simulink model "controllerB_2013B"  (R2013b)
settings: Solver=ode45  StartTime=0.0  StopTime=sim_run  FixedStep=0.001  RelTol=1e-3
InitFcn:
  | zh = 0.01;
undefined symbols (not defined in the file): Standard_Devices, UDP_Protocol, zh_step
libraries: simulink x2, rtwinlib x2, dspnetwork x2
settings Model: Creator=Lenka  LastModifiedBy=Anony
settings DebuggingCC: UnderspecifiedInitializationDetection=Simplified  MergeDetectMultiDrivingBlocksExec=error  FrameProcessingCompatibilityMsg=error
settings GRTTargetCC: CodeReplacementLibrary=C89/C90 (ANSI)

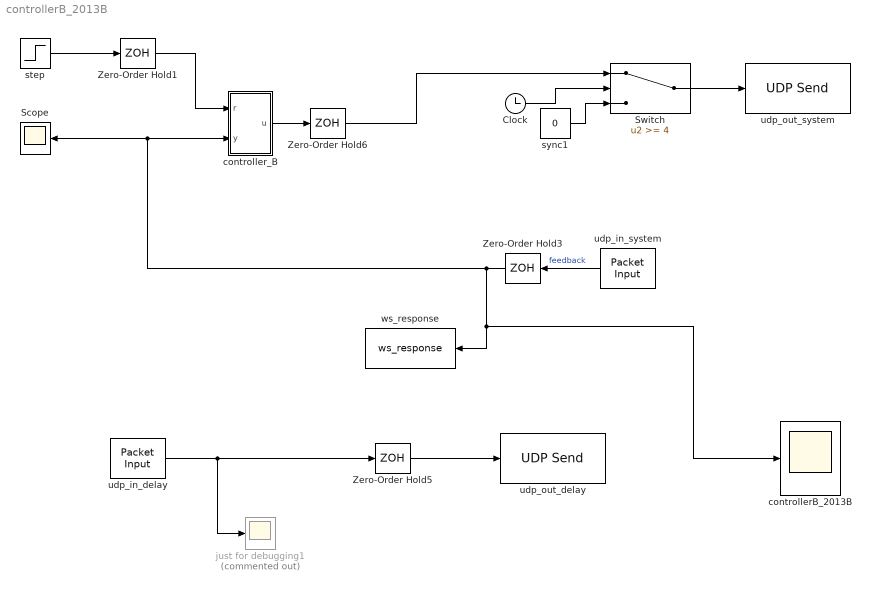
== system controllerB_2013B ==
  Clock : Clock
  Scope : Scope
      settings: YMin=-10  YMax=10
  Switch : Switch  Threshold=4
  Zero-Order Hold{1,3,5..6} (4 alike) : ZeroOrderHold  SampleTime=zh_step
  controllerB_2013B : Scope
      settings: YMin=-1.00000  YMax=1.00000
  controller_B : Subsystem
  just for debugging1 : Scope  Commented=on
      settings: YMin=-10  YMax=10
  step : Step  After=0.15  SampleTime=0
  sync1 : Constant  Value=0
  udp_in_delay : rtwinlib/Packet Input  SampleTime=0.001  MaxMissedTicks=inf  ShowMissedTicks=off  YieldWhenWaiting=off  DrvName=Standard_Devices/UDP_Protocol  DrvAddress=21000  DrvOptions=[2468394757 21000]  PacketSize=8  DataTypes='double'  ShowReady=off  ShowError=off  PacketID=1  ByteOrder=1  ShowTimestamp=off
      settings: AttributesFormatString=Standard Devices\nUDP Protocol [6982h]
  udp_in_system : rtwinlib/Packet Input  SampleTime=0.001  MaxMissedTicks=inf  ShowMissedTicks=off  YieldWhenWaiting=off  DrvName=Standard_Devices/UDP_Protocol  DrvAddress=21500  DrvOptions=[2468394757 21500]  PacketSize=8  DataTypes='double'  ShowReady=off  ShowError=off  PacketID=1  ByteOrder=1  ShowTimestamp=off
      settings: AttributesFormatString=Standard Devices\nUDP Protocol [6F54h]
  udp_out_delay : dspnetwork/UDP Send  remoteURL='147.32.183.5'  remotePort=20000  localURL='0.0.0.0'  localPortSource=Automatically determine  localPort=27000  sampletime=-1  separateLengthPort=0
  udp_out_system : dspnetwork/UDP Send  remoteURL='147.32.183.5'  remotePort=20500  localURL='0.0.0.0'  localPortSource=Automatically determine  localPort=27000  sampletime=-1  separateLengthPort=0
  ws_response : ToWorkspace  VariableName=ws_response  SampleTime=zh_step  SaveFormat=Timeseries
  wires:
  step/1 -> Zero-Order Hold1/1
  udp_in_system/1 -> Zero-Order Hold3/1  "feedback"
  Zero-Order Hold3/1 -> controllerB_2013B/1, ws_response/1, controller_B/2(y), Scope/1
  Zero-Order Hold1/1 -> controller_B/1(r)
  controller_B/1(u) -> Zero-Order Hold6/1
  Switch/1 -> udp_out_system/1
  Zero-Order Hold6/1 -> Switch/1
  Clock/1 -> Switch/2
  sync1/1 -> Switch/3
  udp_in_delay/1 -> just for debugging1/1, Zero-Order Hold5/1
  Zero-Order Hold5/1 -> udp_out_delay/1

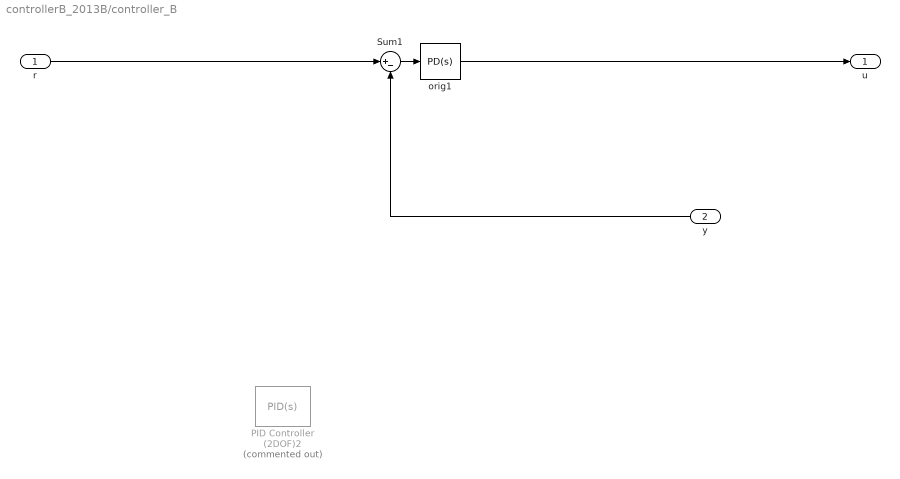
== system controllerB_2013B/controller_B ==
  r : Inport
  y : Inport  Port=2
  PID Controller (2DOF)2 : simulink/Continuous/PID Controller (2DOF)  Commented=on  Controller=PID  TimeDomain=Continuous-time  SampleTime=-1  IntegratorMethod=Forward Euler  FilterMethod=Forward Euler  Form=Parallel  P=6.3799380872686  I=2.12979603411331  D=3.6093223618413  N=48.5068620404972  b=2.39624043732871  c=0.716079145801974  InitialConditionSource=internal  InitialConditionForIntegrator=0  InitialConditionForFilter=0  ExternalReset=none  LimitOutput=off  UpperSaturationLimit=inf  LowerSaturationLimit=-inf  LinearizeAsGain=on  AntiWindupMode=none  Kb=1  TrackingMode=off  Kt=1  PParamMin=[]  PParamMax=[]  IParamMin=[]  IParamMax=[]  DParamMin=[]  DParamMax=[]  NParamMin=[]  NParamMax=[]  bParamMin=[]  bParamMax=[]  cParamMin=[]  cParamMax=[]  KbParamMin=[]  KbParamMax=[]  KtParamMin=[]  KtParamMax=[]  POutMin=[]  POutMax=[]  IOutMin=[]  IOutMax=[]  DOutMin=[]  DOutMax=[]  NOutMin=[]  NOutMax=[]  bOutMin=[]  bOutMax=[]  cOutMin=[]  cOutMax=[]  KbOutMin=[]  KbOutMax=[]  KtOutMin=[]  KtOutMax=[]  IntegratorOutMin=[]  IntegratorOutMax=[]  FilterOutMin=[]  FilterOutMax=[]  SumOutMin=[]  SumOutMax=[]  Sum1OutMin=[]  Sum1OutMax=[]  Sum2OutMin=[]  Sum2OutMax=[]  Sum3OutMin=[]  Sum3OutMax=[]  SumI1OutMin=[]  SumI1OutMax=[]  SumI2OutMin=[]  SumI2OutMax=[]  SumI3OutMin=[]  SumI3OutMax=[]  SumDOutMin=[]  SumDOutMax=[]  SaturationOutMin=[]  SaturationOutMax=[]  IntegratorContinuousStateAttributes=''  IntegratorStateMustResolveToSignalObject=off  IntegratorRTWStateStorageClass=Auto  FilterContinuousStateAttributes=''  FilterStateMustResolveToSignalObject=off  FilterRTWStateStorageClass=Auto
  Sum1 : Sum  Inputs=|+-
  orig1 : simulink/Continuous/PID Controller  Controller=PD  TimeDomain=Continuous-time  SampleTime=-1  IntegratorMethod=Forward Euler  FilterMethod=Forward Euler  Form=Parallel  P=0.0142  I=0.0175856984919557  D=0.0001  N=100  InitialConditionSource=internal  InitialConditionForIntegrator=0  InitialConditionForFilter=0  ExternalReset=none  LimitOutput=on  UpperSaturationLimit=5/1000  LowerSaturationLimit=-5/1000  LinearizeAsGain=on  AntiWindupMode=none  Kb=1  TrackingMode=off  Kt=1  PParamMin=[]  PParamMax=[]  IParamMin=[]  IParamMax=[]  DParamMin=[]  DParamMax=[]  NParamMin=[]  NParamMax=[]  KbParamMin=[]  KbParamMax=[]  KtParamMin=[]  KtParamMax=[]  POutMin=[]  POutMax=[]  IOutMin=[]  IOutMax=[]  DOutMin=[]  DOutMax=[]  NOutMin=[]  NOutMax=[]  KbOutMin=[]  KbOutMax=[]  KtOutMin=[]  KtOutMax=[]  IntegratorOutMin=[]  IntegratorOutMax=[]  FilterOutMin=[]  FilterOutMax=[]  SumOutMin=[]  SumOutMax=[]  SumI1OutMin=[]  SumI1OutMax=[]  SumI2OutMin=[]  SumI2OutMax=[]  SumI3OutMin=[]  SumI3OutMax=[]  SumDOutMin=[]  SumDOutMax=[]  SaturationOutMin=[]  SaturationOutMax=[]  IntegratorContinuousStateAttributes=''  IntegratorStateMustResolveToSignalObject=off  IntegratorRTWStateStorageClass=Auto  FilterContinuousStateAttributes=''  FilterStateMustResolveToSignalObject=off  FilterRTWStateStorageClass=Auto
  u : Outport
  wires:
  orig1/1 -> u/1
  y/1 -> Sum1/2
  r/1 -> Sum1/1
  Sum1/1 -> orig1/1
